simulink model "EV_Powertrain_Modelling"  (R2023a)
settings: Solver=VariableStepAuto  StartTime=0  StopTime=1372  RelTol=1e-3
model workspace (MATLAB code in the model file):
  | Rw = 0.254; % radius of vehicle (m)
  | GVM =330; % Gross vehicle mass (Kg)
  | GVW = GVM*9.81; % Gross vehicle weight (Kg.M/s^2)
  | Crf = 0.015; % Rolling resistance co.efficient
  | Slope_angle = 0; % slope angle-gradient in (rad)
  | Af = 1.1; % Frontal area (m^2)
  | Cd = 0.4; % Drag co.efficient
  | gear_ratio = 6;
  | trans_eff = 0.9; % Transmission efficiency
  | motor_eff = 0.9; % Motor efficiency
  | mc_eff = 0.95; % motor controller efficiency
  | Bv = 72; % Battery voltage (V)
  | Cv = 3.6; % cell voltage - kokum cell (V)
  | Cc = 31; % cell capacity (Ah)
  | lap_distance = 17.77; % distance of one lap (Km)
  | range = 20; % range of vehicle for single charge
  | time = 60; % time required to complete one lap
  | air_density = 1.225; % air density constant
libraries: autolibshared x1
settings Model: Creator=matha  LastModifiedBy=matha

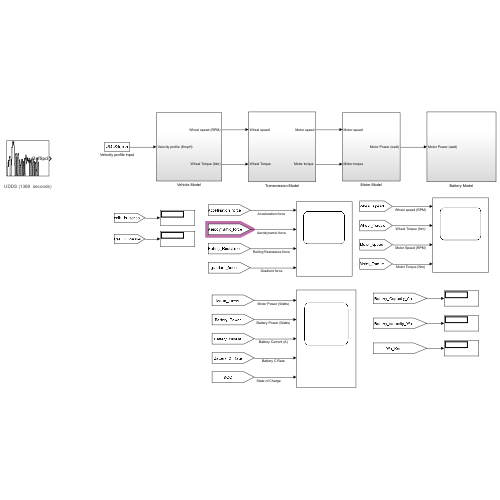
[thumbnail: Simulink's stored preview of the top-level diagram]
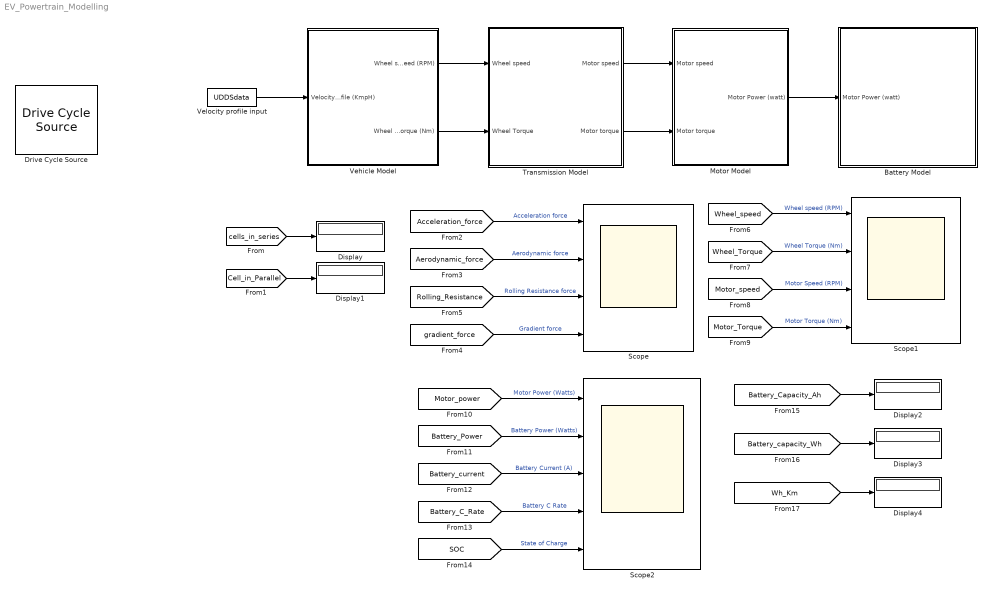
== system EV_Powertrain_Modelling ==
  Battery Model : Subsystem
  Display{,1..4} (5 alike) : Display
      settings: Decimation=2
  Drive Cycle Source : autolibshared/Drive Cycle Source  cycleVar=UDDS  fileVar=cycleFTP75.mat  tfinal="1369  seconds"  cycleRepeat=off  outAccPort=off  outGearPort=off  gearList=No gear data  t_wot1=5  xdot_woto=0  xdot_wot1=30  t_wot2=20  xdot_wot2=0  t_wotend=30  srcUnit=m/s  outUnit=m/s  srcAccUnit=m/s/s  outAccUnit=m/s^2  dt=0  aMode=2  faultOption=off  velBnd=2  velBndUnit=mph  inUnit=m/s  timeBnd=1  failOption=off  stopSim=off  maxFaultCnt=10  maxFaultTime=2  maxTotFaultTime=15  traceOption=off  dtTrace=1  traceWindow=10  lastDCname=FTP75  lastOutUnit=mph  lastDT=0  lastTB=1  lastSB=2  forceCalcBound=off
      settings: LibrarySourceBlock=vdynlib/Vehicle Scenarios/Drive Cycle and Maneuvers/Drive Cycle Source
  Motor Model : Subsystem
  Scope : Scope  NumInputPorts=4
  Scope1 : Scope  NumInputPorts=4
  Scope2 : Scope  NumInputPorts=5
  Transmission Model : Subsystem
  Vehicle Model : Subsystem
  Velocity profile input : FromWorkspace  VariableName=UDDSdata
  wires:
  Vehicle Model/1(Wheel speed (RPM)) -> Transmission Model/1(Wheel speed)
  Vehicle Model/2(Wheel Torque (Nm)) -> Transmission Model/2(Wheel Torque)
  Transmission Model/1(Motor speed) -> Motor Model/1(Motor speed)
  Transmission Model/2("Motor torque ") -> Motor Model/2(Motor torque)
  Motor Model/1(Motor Power (watt)) -> Battery Model/1(Motor Power (watt))
  [cells_in_series] -> Display/1
  [Cell_in_Parallel] -> Display1/1
  [gradient_force] -> Scope/4  "Gradient force"
  [Rolling_Resistance] -> Scope/3  "Rolling Resistance force"
  [Aerodynamic_force] -> Scope/2  "Aerodynamic force"
  [Acceleration_force] -> Scope/1  "Acceleration force"
  [Wheel_speed] -> Scope1/1  "Wheel speed (RPM)"
  [Wheel_Torque] -> Scope1/2  "Wheel Torque (Nm)"
  [Motor_speed] -> Scope1/3  "Motor Speed (RPM)"
  [Motor_Torque] -> Scope1/4  "Motor Torque (Nm)"
  [Battery_Power] -> Scope2/2  "Battery Power (Watts)"
  [Battery_C_Rate] -> Scope2/4  "Battery C Rate"
  [Battery_current] -> Scope2/3  "Battery Current (A)"
  [Motor_power] -> Scope2/1  "Motor Power (Watts)"
  [SOC] -> Scope2/5  "State of Charge"
  [Battery_Capacity_Ah] -> Display2/1
  [Battery_capacity_Wh] -> Display3/1
  [Wh_Km] -> Display4/1
  Velocity profile input/1 -> Vehicle Model/1(Velocity profile (KmpH))

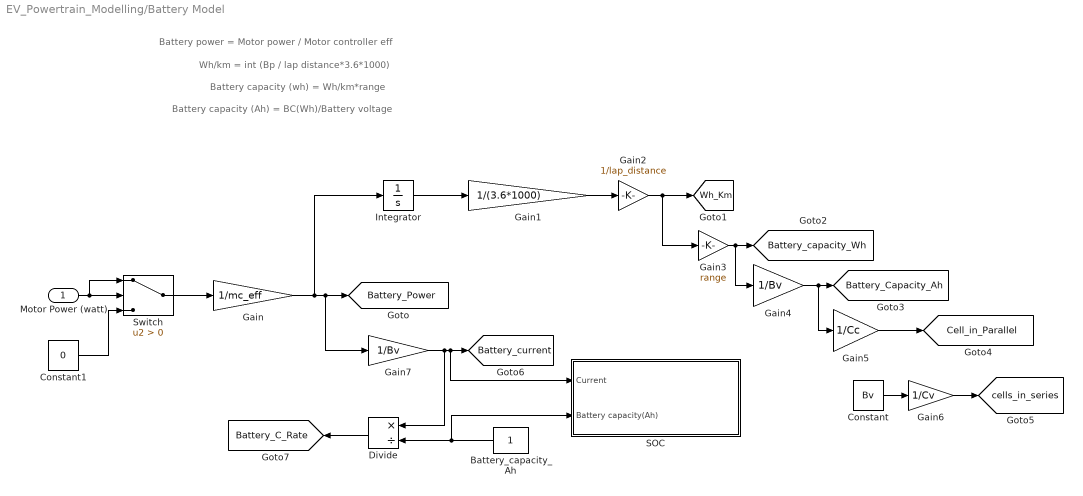
== system EV_Powertrain_Modelling/Battery Model ==
  note: Battery capacity (Ah) = BC(Wh)/Battery voltage
  note: Battery capacity (wh) = Wh/km*range
  note: Wh/km = int (Bp / lap distance*3.6*1000)
  note: Battery power = Motor power / Motor controller eff
  Motor Power (watt) : Inport
  Battery_capacity_Ah : Constant
  Constant : Constant  Value=Bv
  Constant1 : Constant  Value=0
  Divide : Product  Inputs=*/
  Gain : Gain  Gain=1/mc_eff
  Gain1 : Gain  Gain=1/(3.6*1000)
  Gain2 : Gain  Gain=1/lap_distance
  Gain3 : Gain  Gain=range
  Gain4 : Gain  Gain=1/Bv
  Gain5 : Gain  Gain=1/Cc
  Gain6 : Gain  Gain=1/Cv
  Gain7 : Gain  Gain=1/Bv
  Integrator : Integrator
  SOC : Subsystem
  Switch : Switch  Criteria=u2 > Threshold  SaturateOnIntegerOverflow=off  InputSameDT=off
  tag scope: Battery_C_Rate=global, Battery_Capacity_Ah=global, Battery_Power=global, Battery_capacity_Wh=global, Battery_current=global, Cell_in_Parallel=global, Wh_Km=global, cells_in_series=global
  wires:
  Motor Power (watt)/1 -> Switch/1, Switch/2
  Constant1/1 -> Switch/3
  Switch/1 -> Gain/1
  Gain/1 -> Integrator/1, Gain7/1, [Battery_Power]
  Integrator/1 -> Gain1/1
  Gain1/1 -> Gain2/1
  Gain2/1 -> Gain3/1, [Wh_Km]
  Gain3/1 -> Gain4/1, [Battery_capacity_Wh]
  Gain4/1 -> Gain5/1, [Battery_Capacity_Ah]
  Gain5/1 -> [Cell_in_Parallel]
  Constant/1 -> Gain6/1
  Gain6/1 -> [cells_in_series]
  Gain7/1 -> Divide/1, SOC/1(Current), [Battery_current]
  Battery_capacity_Ah/1 -> SOC/2(Battery capacity(Ah)), Divide/2
  Divide/1 -> [Battery_C_Rate]

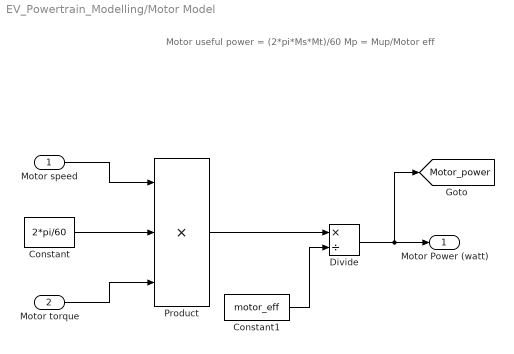
== system EV_Powertrain_Modelling/Motor Model ==
  note: Motor useful power = (2*pi*Ms*Mt)/60
      | Mp = Mup/Motor eff
  Motor speed : Inport
  Motor torque : Inport  Port=2
  Constant : Constant  Value=2*pi/60
  Constant1 : Constant  Value=motor_eff
  Divide : Product  Inputs=*/
  Product : Product  Inputs=3
  Motor Power (watt) : Outport
  tag scope: Motor_power=global
  wires:
  Constant/1 -> Product/2
  Motor speed/1 -> Product/1
  Motor torque/1 -> Product/3
  Product/1 -> Divide/1
  Constant1/1 -> Divide/2
  Divide/1 -> [Motor_power], Motor Power (watt)/1

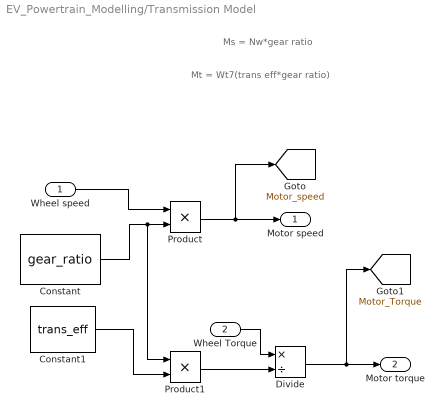
== system EV_Powertrain_Modelling/Transmission Model ==
  note: Mt = Wt7(trans eff*gear ratio)
  note: Ms = Nw*gear ratio
  Wheel speed : Inport
  Wheel Torque : Inport  Port=2
  Constant : Constant  Value=gear_ratio
  Constant1 : Constant  Value=trans_eff
  Divide : Product  Inputs=*/
  Product : Product
  Product1 : Product
  Motor speed : Outport
  "Motor torque " : Outport  Port=2
  tag scope: Motor_Torque=global, Motor_speed=global
  wires:
  Wheel speed/1 -> Product/1
  Constant/1 -> Product1/1, Product/2
  Product/1 -> [Motor_speed], Motor speed/1
  Constant1/1 -> Product1/2
  Wheel Torque/1 -> Divide/1
  Product1/1 -> Divide/2
  Divide/1 -> [Motor_Torque], "Motor torque "/1

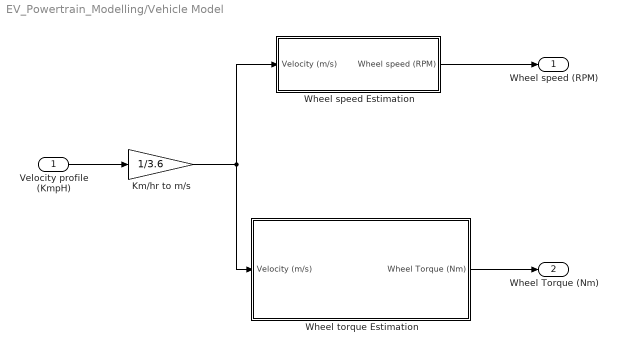
== system EV_Powertrain_Modelling/Vehicle Model ==
  Velocity profile (KmpH) : Inport
  Km/hr to m/s : Gain  Gain=1/3.6
  Wheel speed Estimation : Subsystem
  Wheel torque Estimation : Subsystem
  Wheel speed (RPM) : Outport
  Wheel Torque (Nm) : Outport  Port=2
  wires:
  Velocity profile (KmpH)/1 -> Km/hr to m/s/1
  Km/hr to m/s/1 -> Wheel speed Estimation/1(Velocity (m/s)), Wheel torque Estimation/1(Velocity (m/s))
  Wheel speed Estimation/1(Wheel speed (RPM)) -> Wheel speed (RPM)/1
  Wheel torque Estimation/1(Wheel Torque (Nm)) -> Wheel Torque (Nm)/1

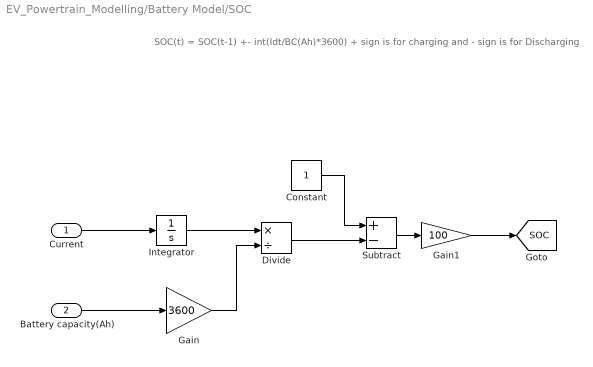
== system EV_Powertrain_Modelling/Battery Model/SOC ==
  note: SOC(t) = SOC(t-1) +- int(Idt/BC(Ah)*3600)
      | + sign is for charging and - sign is for Discharging
  Current : Inport
  Battery capacity(Ah) : Inport  Port=2
  Constant : Constant
  Divide : Product  Inputs=*/
  Gain : Gain  Gain=3600
  Gain1 : Gain  Gain=100
  Integrator : Integrator
  Subtract : Sum  Inputs=+-
  tag scope: SOC=global
  wires:
  Battery capacity(Ah)/1 -> Gain/1
  Current/1 -> Integrator/1
  Integrator/1 -> Divide/1
  Gain/1 -> Divide/2
  Divide/1 -> Subtract/2
  Constant/1 -> Subtract/1
  Subtract/1 -> Gain1/1
  Gain1/1 -> [SOC]

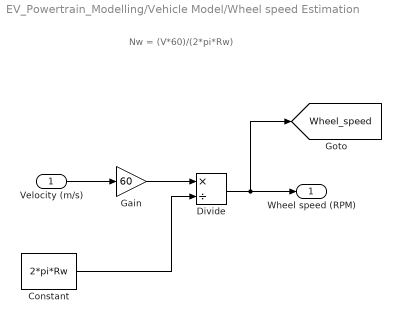
== system EV_Powertrain_Modelling/Vehicle Model/Wheel speed Estimation ==
  note: Nw = (V*60)/(2*pi*Rw)
  Velocity (m/s) : Inport
  Constant : Constant  Value=2*pi*Rw
  Divide : Product  Inputs=*/
  Gain : Gain  Gain=60
  Wheel speed (RPM) : Outport
  tag scope: Wheel_speed=global
  wires:
  Velocity (m/s)/1 -> Gain/1
  Gain/1 -> Divide/1
  Constant/1 -> Divide/2
  Divide/1 -> [Wheel_speed], Wheel speed (RPM)/1

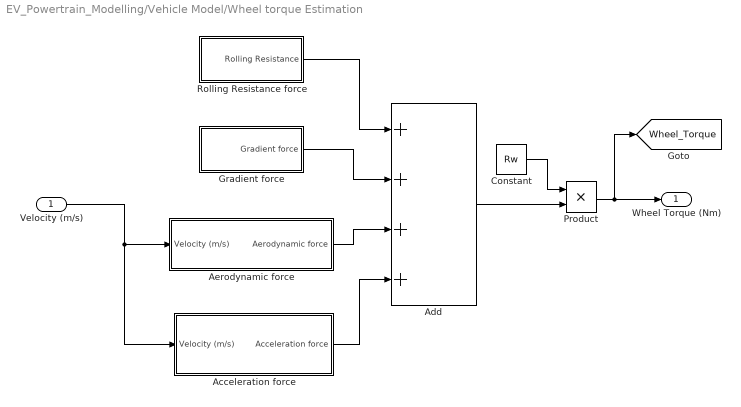
== system EV_Powertrain_Modelling/Vehicle Model/Wheel torque Estimation ==
  Velocity (m/s) : Inport
  Acceleration force : Subsystem
  Add : Sum  Inputs=++++
  Aerodynamic force : Subsystem
  Constant : Constant  Value=Rw
  Gradient force : Subsystem
  Product : Product
  Rolling Resistance force : Subsystem
  Wheel Torque (Nm) : Outport
  tag scope: Wheel_Torque=global
  wires:
  Rolling Resistance force/1(Rolling Resistance) -> Add/1
  Gradient force/1(Gradient force) -> Add/2
  Aerodynamic force/1(Aerodynamic force) -> Add/3
  Acceleration force/1(Acceleration force) -> Add/4
  Velocity (m/s)/1 -> Acceleration force/1(Velocity (m/s)), Aerodynamic force/1(Velocity (m/s))
  Add/1 -> Product/2
  Constant/1 -> Product/1
  Product/1 -> [Wheel_Torque], Wheel Torque (Nm)/1

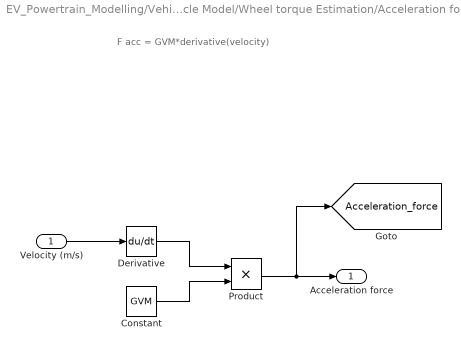
== system EV_Powertrain_Modelling/Vehicle Model/Wheel torque Estimation/Acceleration force ==
  note: F acc = GVM*derivative(velocity)
  Velocity (m/s) : Inport
  Constant : Constant  Value=GVM
  Derivative : Derivative
  Product : Product
  Acceleration force : Outport
  tag scope: Acceleration_force=global
  wires:
  Velocity (m/s)/1 -> Derivative/1
  Derivative/1 -> Product/1
  Constant/1 -> Product/2
  Product/1 -> [Acceleration_force], Acceleration force/1

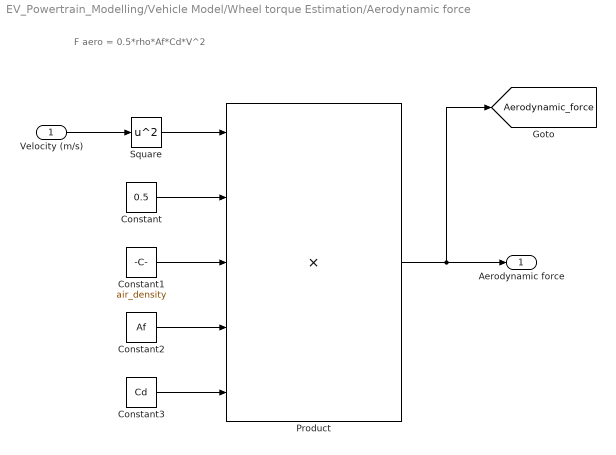
== system EV_Powertrain_Modelling/Vehicle Model/Wheel torque Estimation/Aerodynamic force ==
  note: F aero = 0.5*rho*Af*Cd*V^2
  Velocity (m/s) : Inport
  Constant : Constant  Value=0.5
  Constant1 : Constant  Value=air_density
  Constant2 : Constant  Value=Af
  Constant3 : Constant  Value=Cd
  Product : Product  Inputs=5
  Square : Math  Operator=square
  Aerodynamic force : Outport
  tag scope: Aerodynamic_force=global
  wires:
  Velocity (m/s)/1 -> Square/1
  Square/1 -> Product/1
  Constant/1 -> Product/2
  Constant1/1 -> Product/3
  Constant2/1 -> Product/4
  Constant3/1 -> Product/5
  Product/1 -> [Aerodynamic_force], Aerodynamic force/1

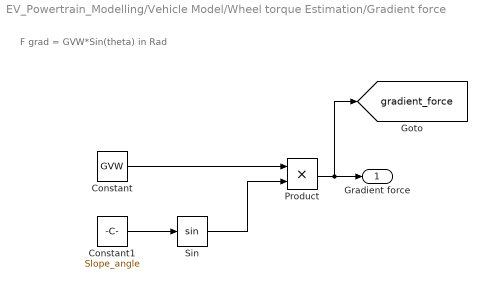
== system EV_Powertrain_Modelling/Vehicle Model/Wheel torque Estimation/Gradient force ==
  note: F grad = GVW*Sin(theta) in Rad
  Constant : Constant  Value=GVW
  Constant1 : Constant  Value=Slope_angle
  Product : Product
  Sin : Trigonometry
  Gradient force : Outport
  tag scope: gradient_force=global
  wires:
  Constant1/1 -> Sin/1
  Constant/1 -> Product/1
  Sin/1 -> Product/2
  Product/1 -> [gradient_force], Gradient force/1

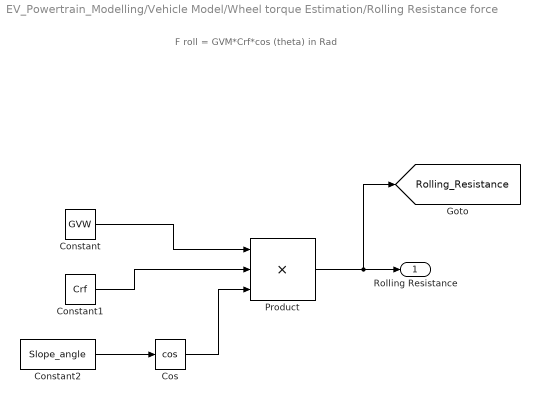
== system EV_Powertrain_Modelling/Vehicle Model/Wheel torque Estimation/Rolling Resistance force ==
  note: F roll = GVM*Crf*cos (theta)
      | in Rad
  Constant : Constant  Value=GVW
  Constant1 : Constant  Value=Crf
  Constant2 : Constant  Value=Slope_angle
  Cos : Trigonometry  Operator=cos
  Product : Product  Inputs=3
  Rolling Resistance : Outport
  tag scope: Rolling_Resistance=global
  wires:
  Constant/1 -> Product/1
  Constant1/1 -> Product/2
  Constant2/1 -> Cos/1
  Cos/1 -> Product/3
  Product/1 -> [Rolling_Resistance], Rolling Resistance/1
